simulink model "kouz1"  (R2021a)
settings: Solver=FixedStepDiscrete  StartTime=0.0  StopTime=128  RelTol=1e-3
libraries: dspsrcs4 x1, dspxfrm3 x1
settings Model: Creator=User1  LastModifiedBy=User1
settings SolverCC: AlgebraicLoopSolver=TrustRegion
settings DataIOCC: LimitDataPoints=on  SaveOutput=off  SignalLogging=off  SaveTime=off
settings OptimizationCC: LifeSpan=inf  SimCompilerOptimization=on
settings DebuggingCC: AlgebraicLoopMsg=error  SingleTaskRateTransMsg=error  AllowSymbolicDim=off  SFUnexpectedBacktrackingDiag=warning  SFNoUnconditionalDefaultTransitionDiag=warning  SFExecutionAtInitializationDiag=none  SFMachineParentedDataDiag=warning  ArithmeticOperatorsInVariantConditions=warning
settings SFSimCC: SimUseLocalCustomCode=off  CustomCodeUndefinedFunction=UseInterfaceOnly
settings RTWCC: RTWUseLocalCustomCode=off
settings CodeAppCC: StateflowObjectComments=on
settings GRTTargetCC: TargetLangStandard=C89/C90 (ANSI)
settings ConfigComp: CovMetricSettings=dw  CovSaveCumulativeToWorkspaceVar=on  CovSaveSingleToWorkspaceVar=on  CovExternalEMLEnable=off  CovSFcnEnable=off

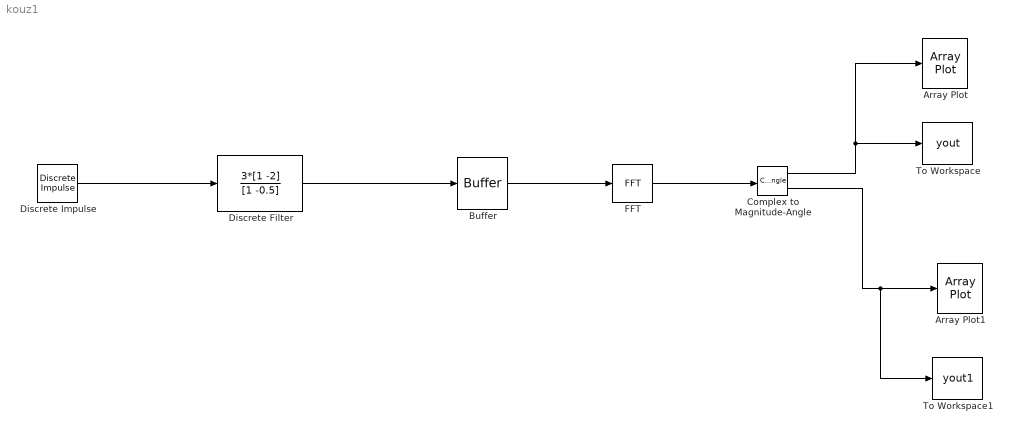
== system kouz1 ==
  Array Plot : ArrayPlot  WindowPosition=[368.000000,182.000000,800.000000,500.000000,]  DefaultConfigurationName=dsp.scopes.ArrayPlotBlockSpecification
  Array Plot1 : ArrayPlot  WindowPosition=[463.000000,128.000000,800.000000,500.000000,]  DefaultConfigurationName=dsp.scopes.ArrayPlotBlockSpecification
  Buffer : Buffer  N=128  OutputFrames=off
  Complex to Magnitude-Angle : ComplexToMagnitudeAngle
  Discrete Impulse : dspsrcs4/Discrete  Impulse  Delay=0  SampleTime=1  FrameSample=1  OutputFrames=off  dataType=double  isSigned=on  wordLen=16  udDataType=sfix(16)  fracBitsMode=Best precision  numFracBits=15  OutDataTypeStr=double  LastOutDataTypeStr=double
  Discrete Filter : DiscreteFilter  Numerator=3*[1 -2]  Denominator=[1 -0.5]  InputProcessing=Columns as channels (frame based)  FilterStructure=Direct form II transposed  a0EqualsOne=on
  FFT : dspxfrm3/FFT  FFTImplementation=Auto  CompMethod=Table lookup  TableOpt=NEW  TableOptActive=Speed  BitRevOrder=off  Normalize=off  InheritFFTLength=on  FFTLength=64  WrapInput=on  roundingMode=Floor  overflowMode=off  firstCoeffDataTypeStr=Inherit: Same word length as input  firstCoeffLastDataTypeStr=Inherit: Same word length as input  outputMin=[]  outputMax=[]
  To Workspace : ToWorkspace  VariableName=yout  SampleTime=-1
      settings: Save2DSignal=2-D array (concatenate along first dimension)
  To Workspace1 : ToWorkspace  VariableName=yout1  SampleTime=-1
      settings: Save2DSignal=2-D array (concatenate along first dimension)
  wires:
  Discrete Filter/1 -> Buffer/1
  Discrete Impulse/1 -> Discrete Filter/1
  FFT/1 -> Complex to Magnitude-Angle/1
  Buffer/1 -> FFT/1
  Complex to Magnitude-Angle/1 -> To Workspace/1, Array Plot/1
  Complex to Magnitude-Angle/2 -> To Workspace1/1, Array Plot1/1
